simulink model "SIM5"  (R2021a)
settings: Solver=VariableStepAuto  StartTime=0.0  StopTime=100  RelTol=1e-3
settings Model: Creator=jmata  LastModifiedBy=jmata

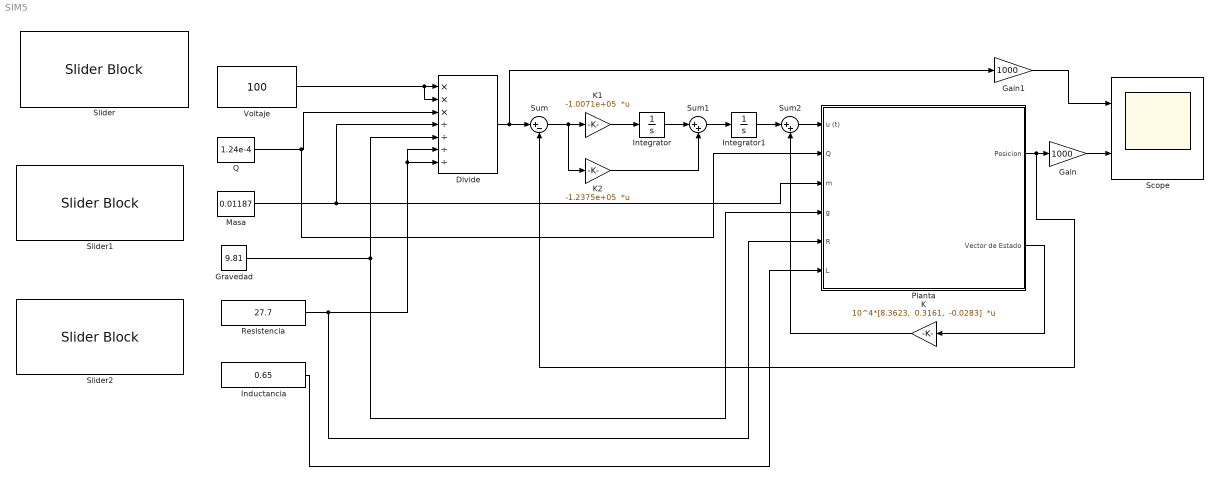
== system SIM5 ==
  Divide : Product  Inputs=***////
  Gain : Gain  Gain=1000
  Gain1 : Gain  Gain=1000
  Gravedad : Constant  Value=9.81
  Inductancia : Constant  Value=0.65
  Integrator : Integrator
  Integrator1 : Integrator
  K : Gain  Gain="10^4*[8.3623,  0.3161,  -0.0283]"  Multiplication=Matrix(K*u)
  K1 : Gain  Gain=-1.0071e+05  Multiplication=Matrix(K*u)
  K2 : Gain  Gain=-1.2375e+05  Multiplication=Matrix(K*u)
  Masa : Constant  Value=0.01187
  Planta : Subsystem
  Q : Constant  Value=1.24e-4
  Resistencia : Constant  Value=27.7
  Scope : Scope  NumInputPorts=2
  Slider : SliderBlock  ScaleMin=99  ScaleMax=121
  Slider1 : SliderBlock  ScaleMin=25  ScaleMax=30
  Slider2 : SliderBlock  ScaleMin=0.585  ScaleMax=0.715
  Sum : Sum  Inputs=|+-
  Sum1 : Sum  Inputs=|++
  Sum2 : Sum  Inputs=|++
  Voltaje : Constant  Value=100
  wires:
  Voltaje/1 -> Divide/2, Divide/1
  Q/1 -> Planta/2(Q), Divide/3
  Masa/1 -> Planta/3(m), Divide/4
  Gravedad/1 -> Divide/5, Planta/4(g)
  Resistencia/1 -> Divide/7, Divide/6, Planta/5(R)
  Divide/1 -> Gain1/1, Sum/1
  Sum/1 -> K2/1, K1/1
  K1/1 -> Integrator/1
  Integrator/1 -> Sum1/1
  K2/1 -> Sum1/2
  Sum1/1 -> Integrator1/1
  Integrator1/1 -> Sum2/1
  Sum2/1 -> Planta/1(u (t))
  Planta/1(Posicion) -> Gain/1, Sum/2
  Gain/1 -> Scope/2
  Planta/2(Vector de Estado) -> K/1
  K/1 -> Sum2/2
  Inductancia/1 -> Planta/6(L)
  Gain1/1 -> Scope/1

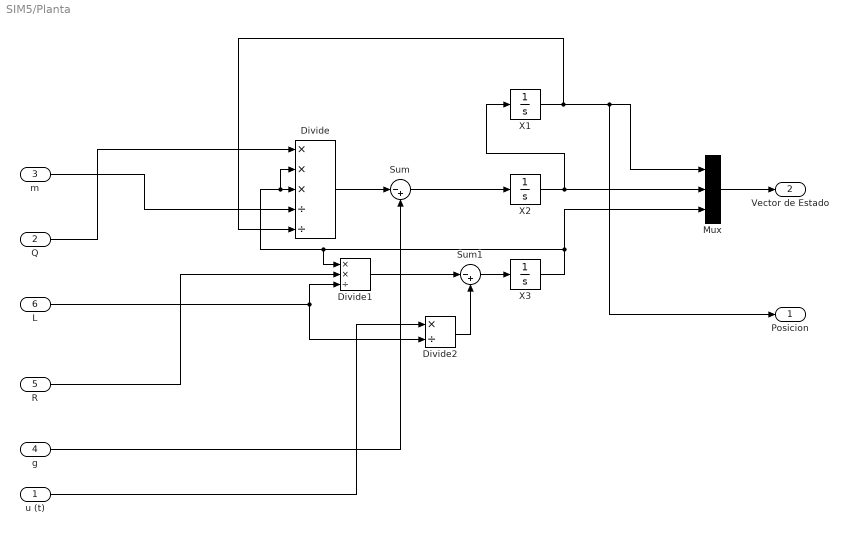
== system SIM5/Planta ==
  u (t) : Inport
  Q : Inport  Port=2
  m : Inport  Port=3
  g : Inport  Port=4
  R : Inport  Port=5
  L : Inport  Port=6
  Divide : Product  Inputs=***//
  Divide1 : Product  Inputs=**/
  Divide2 : Product  Inputs=*/
  Mux : Mux  Inputs=3
  Sum : Sum  Inputs=|-+
  Sum1 : Sum  Inputs=|-+
  X1 : Integrator  InitialCondition=0.01
  X2 : Integrator
  X3 : Integrator  InitialCondition=3
  Posicion : Outport
  Vector de Estado : Outport  Port=2
  wires:
  Divide/1 -> Sum/1
  Sum/1 -> X2/1
  L/1 -> Divide2/2, Divide1/3
  Sum1/1 -> X3/1
  X3/1 -> Mux/3, Divide1/1, Divide/2, Divide/3
  Divide2/1 -> Sum1/2
  X1/1 -> Posicion/1, Mux/1, Divide/5
  X2/1 -> Mux/2, X1/1
  g/1 -> Sum/2
  Divide1/1 -> Sum1/1
  m/1 -> Divide/4
  Q/1 -> Divide/1
  Mux/1 -> Vector de Estado/1
  R/1 -> Divide1/2
  u (t)/1 -> Divide2/1
